simulink model "Ejercicio_1_DB_PID"  (R2023a)
settings: Solver=VariableStepAuto  StartTime=0.0  StopTime=150  RelTol=1e-6
values from neighbouring files (symbols this model uses):
  A = 10    [Ejercicio_1.m]    (also in Ejercicio_2y3.m)
  A1 = 1e-2    (= 0.01)    [Ejercicio_1.m]    (also in Ejercicio_2y3.m)
  A2 = 1    [Ejercicio_1.m]    (also in Ejercicio_2y3.m)
  bT = bm + (R*A1)^2*Rh + (R*A1/A2)^2*bp    (= 6.227045)    [Ejercicio_1.m]    (also in Ejercicio_2y3.m)
  JT = Jm + Jr + R^2*mp + (R*A1/A2)^2*m    (= 4.5108)    [Ejercicio_1.m]    (also in Ejercicio_2y3.m)
  K_D = 350    [Ejercicio_1.m]
  K_I = K_D * NGc(3)    [Ejercicio_1.m]
  K_P = K_D * NGc(2)    [Ejercicio_1.m]
  Kb = 1    [Ejercicio_1.m]    (also in Ejercicio_2y3.m)
  kP = 5    [Ejercicio_1.m]    (also in Ejercicio_2y3.m)
  Kt = 1    [Ejercicio_1.m]    (also in Ejercicio_2y3.m)
  kT = (R*A1)^2/Ch + (R*A1/A2)^2*km    (= 0.26829)    [Ejercicio_1.m]    (also in Ejercicio_2y3.m)
  La = 100e-3    (= 0.1)    [Ejercicio_1.m]    (also in Ejercicio_2y3.m)
  R = 0.3    [Ejercicio_1.m]    (also in Ejercicio_2y3.m)
  Ra = 2.1    [Ejercicio_1.m]    (also in Ejercicio_2y3.m)
  VR = 10    [Ejercicio_1.m]
libraries: slpidlib x1
settings Model: Creator=54115  LastModifiedBy=franc
settings SolverCC: AlgebraicLoopSolver=TrustRegion
settings DebuggingCC: UnconnectedInputMsg=warning  UnconnectedOutputMsg=warning  UnconnectedLineMsg=warning
settings ModelReferenceCC: EnableRefExpFcnMdlSchedulingChecks=on

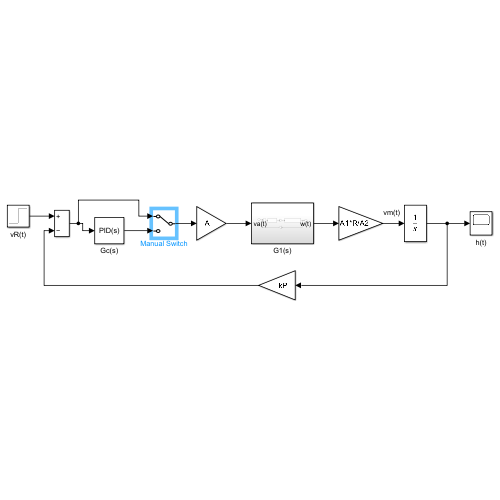
[thumbnail: Simulink's stored preview of the top-level diagram]
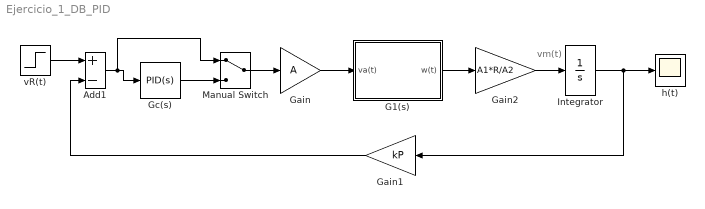
== system Ejercicio_1_DB_PID ==
  note: vm(t)
  Add1 : Sum  Inputs=+-
  G1(s) : Subsystem
  Gain : Gain  Gain=A
  Gain1 : Gain  Gain=kP
  Gain2 : Gain  Gain=A1*R/A2
  Gc(s) : slpidlib/PID Controller  Controller=PID  Form=Parallel  TimeDomain=Continuous-time  UseExternalTs=off  SampleTime=-1  IntegratorMethod=Forward Euler  FilterMethod=Forward Euler  ControllerParametersSource=internal  P=K_P  I=K_I  UseKiTs=off  D=K_D  N=100  UseFilter=on  TunerSelectOption=Transfer Function Based (PID Tuner App)  InitialConditionSource=internal  InitialConditionForIntegrator=0  InitialConditionForFilter=0  DifferentiatorICPrevScaledInput=0  ExternalReset=none  TrackingMode=off  Kt=1  LimitOutput=off  SatLimitsSource=internal  UpperSaturationLimit=inf  LowerSaturationLimit=-inf  LinearizeAsGain=on  AntiWindupMode=none  Kb=1  LimitIntegrator=off  UpperIntegratorSaturationLimit=inf  LowerIntegratorSaturationLimit=-inf  POutMin=[]  POutMax=[]  IOutMin=[]  IOutMax=[]  DOutMin=[]  DOutMax=[]  NOutMin=[]  NOutMax=[]  SumOutMin=[]  SumOutMax=[]  SaturationOutMin=[]  SaturationOutMax=[]  PParamMin=[]  PParamMax=[]  IParamMin=[]  IParamMax=[]  DParamMin=[]  DParamMax=[]  NParamMin=[]  NParamMax=[]  KbParamMin=[]  KbParamMax=[]  KtParamMin=[]  KtParamMax=[]  KbOutMin=[]  KbOutMax=[]  KtOutMin=[]  KtOutMax=[]  IntegratorOutMin=[]  IntegratorOutMax=[]  FilterOutMin=[]  FilterOutMax=[]  SumI1OutMin=[]  SumI1OutMax=[]  SumI2OutMin=[]  SumI2OutMax=[]  SumI3OutMin=[]  SumI3OutMax=[]  SumI4OutMin=[]  SumI4OutMax=[]  SumDOutMin=[]  SumDOutMax=[]  DifferentiatorOutMin=[]  DifferentiatorOutMax=[]  FilterDiffOutCoefMin=[]  FilterDiffOutCoefMax=[]  ReciprocalOutMin=[]  ReciprocalOutMax=[]  SumDenOutMin=[]  SumDenOutMax=[]  SumNumOutMin=[]  SumNumOutMax=[]  DivideOutMin=[]  DivideOutMax=[]  UdiffTsProdOutMin=[]  UdiffTsProdOutMax=[]  NTsProdOutMin=[]  NTsProdOutMax=[]  UintegralTsProdOutMin=[]  UintegralTsProdOutMax=[]  UngainTsProdOutMin=[]  UngainTsProdOutMax=[]  ClampingZeroOutDataTypeStr=Inherit: Inherit via back propagation  ClampingZeroOutMin=[]  ClampingZeroOutMax=[]  FilterDenConstantOutDataTypeStr=Inherit: Inherit via back propagation  FilterDenConstantOutMin=[]  FilterDenConstantOutMax=[]  PCopyOutDataTypeStr=Inherit: Inherit via back propagation  PCopyOutMin=[]  PCopyOutMax=[]  NCopyOutDataTypeStr=Inherit: Inherit via back propagation  NCopyOutMin=[]  NCopyOutMax=[]  IntegratorContinuousStateAttributes=''  IntegratorStateMustResolveToSignalObject=off  IntegratorRTWStateStorageClass=Auto  FilterContinuousStateAttributes=''  FilterStateMustResolveToSignalObject=off  FilterRTWStateStorageClass=Auto  ParallelPVariant=InternalParameters  IdealPVariant=Disabled  IVariant=InternalParameters  DVariant=InternalParameters  IntegratorVariant=Continuous  SatVariant=Disabled  AWVariant=Passthrough  PCopyVariant=Disabled  TRVariant=Disabled  FdbkBlocksVariant=Forward  IdealPFdbkVariant=Disabled  SatFdbkVariant=Disabled  DerivativeFilterVariant=ContFilter  NVariant=InternalParameters  NCopyVariant=Disabled  FilterICVariant=InternalICsFilter  IntegratorICVariant=InternalICs  ExternalResetVariant=Disabled  TRSumVariant=Passthrough  SumFdbkVariant=Disabled  SumVariant=Sum_PID  TsampFilterVariant=InternalTs  TsampNgainVariant=Passthrough  TsampIntegralVariant=Disabled_SignalSpec  ExternalSaturationOutDataTypeStr=Inherit: Same as second input
  Integrator : Integrator
  Manual Switch : ManualSwitch
  h(t) : Scope
  vR(t) : Step  Time=0  After=VR  SampleTime=0
  wires:
  vR(t)/1 -> Add1/1
  Gain1/1 -> Add1/2
  Gain/1 -> G1(s)/1(va(t))
  G1(s)/1(w(t)) -> Gain2/1
  Gain2/1 -> Integrator/1
  Integrator/1 -> h(t)/1, Gain1/1
  Manual Switch/1 -> Gain/1
  Add1/1 -> Manual Switch/1, Gc(s)/1
  Gc(s)/1 -> Manual Switch/2

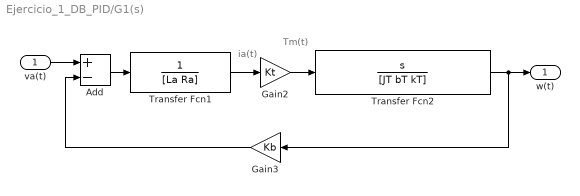
== system Ejercicio_1_DB_PID/G1(s) ==
  note: ia(t)
  note: Tm(t)
  va(t) : Inport
  Add : Sum  Inputs=+-
  Gain2 : Gain  Gain=Kt
  Gain3 : Gain  Gain=Kb
  Transfer Fcn1 : TransferFcn  Denominator=[La Ra]
  Transfer Fcn2 : TransferFcn  Numerator=[1 0]  Denominator=[JT bT kT]
  w(t) : Outport
  wires:
  Gain2/1 -> Transfer Fcn2/1
  Add/1 -> Transfer Fcn1/1
  Gain3/1 -> Add/2
  va(t)/1 -> Add/1
  Transfer Fcn2/1 -> w(t)/1, Gain3/1
  Transfer Fcn1/1 -> Gain2/1
